simulink model "ADAPT_mpc"  (R2021a)
settings: Solver=VariableStepAuto  StartTime=0.0  StopTime=10.0  RelTol=1e-3
values from neighbouring files (symbols this model uses):
  A = [-0.0136411            0.240871                   0               -9.81 ... (first row only)    [MPC_controller_adapt.m]
  B = [ 0.9058396 2 ... (first row only)    [MPC_controller_adapt.m]
  C = [0 1 0 0;0 0 0 1]    [MPC_controller_adapt.m]
  D = [0 0;0 0]    [MPC_controller_adapt.m]
libraries: mpclib x1, cstblocks x1
settings Model: Creator=astik  LastModifiedBy=astik

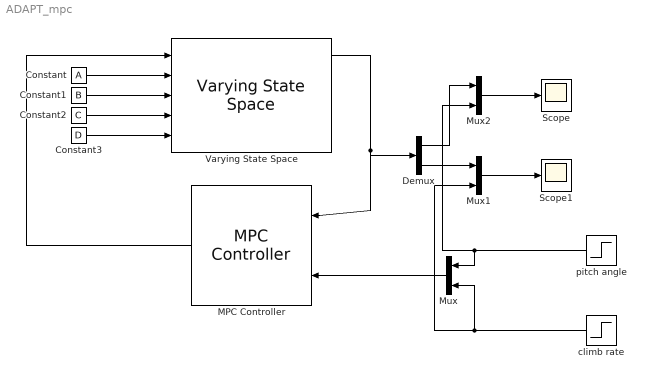
== system ADAPT_mpc ==
  Constant : Constant  Value=A
  Constant1 : Constant  Value=B
  Constant2 : Constant  Value=C
  Constant3 : Constant  Value=D
  Demux : Demux  Outputs=2
  MPC Controller : mpclib/MPC Controller  SCDEnableBlockLinearizationSpecification=on  mpcobj=mpcobj  is_multiple=0  enable_value=0  return_u0=off  updateMPCinCallerWorkspace=on  md_inport=off  mv_inport=off  uref_inport=off  return_cost=off  return_mvseq=off  return_qpstatus=off  return_xseq=off  return_state=off  return_ovseq=off  state_inport=off  umin_inport=off  umax_inport=off  ymin_inport=off  ymax_inport=off  cc_inport=off  ywt_inport=off  uwt_inport=off  duwt_inport=off  rhoeps_inport=off  pm_inport=off  MaximumP=10  HorizonChoice=FixedHorizon  n_ts=0.05  n_p=10  n_mv=2  n_md=0  n_ud=0  n_mo=2  n_uo=0  BlockDataType=double  SampleTimeInherited=off  switch_inport=off
  Mux : Mux  Inputs=2
  Mux1 : Mux  Inputs=2
  Mux2 : Mux  Inputs=2
  Scope : Scope
  Scope1 : Scope
  Varying State Space : cstblocks/Linear Parameter Varying/Varying State Space  x0=0  xNames=''  OutputX=on  OutputDX=on
  climb rate : Step  After=0  SampleTime=0
  pitch angle : Step  After=3  SampleTime=0
  wires:
  MPC Controller/1 -> Varying State Space/1
  Varying State Space/1 -> MPC Controller/1, Demux/1
  Constant/1 -> Varying State Space/2
  Constant3/1 -> Varying State Space/5
  Constant2/1 -> Varying State Space/4
  Constant1/1 -> Varying State Space/3
  Mux/1 -> MPC Controller/2
  pitch angle/1 -> Mux2/2, Mux/1
  climb rate/1 -> Mux1/2, Mux/2
  Demux/2 -> Mux1/1
  Mux1/1 -> Scope1/1
  Mux2/1 -> Scope/1
  Demux/1 -> Mux2/1
